simulink model "AMR_main_24a_TesteMobotic"  (R2024a)
settings: Solver=FixedStepAuto  StartTime=0.0  StopTime=inf  FixedStep=1e-3  RelTol=1e-3
model workspace (MAT data in the model file):
  RTK_health_condition = 30
  mdlWSDbList : string (value not decoded)
undefined symbols (not defined in the file or in its folder): Down, Pull
libraries: tramontina_database_nvidialib x11, speedgoatlib_IO60X_IO69X x10, tramontina_database_curtislib x7, tramontina_database_xsenslib x4, tramontina_database_moboticlib x2, speedgoatlib_IO691 x2, canmsglib x1
(part 2 of 2)

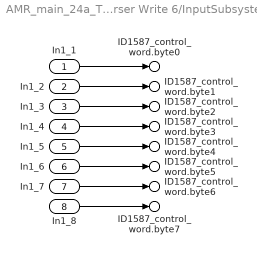
== system AMR_main_24a_TesteMobotic/CAN DB Parser Write 6/InputSubsystem ==
  In1_1 : Inport
  In1_2 : Inport  Port=2
  In1_3 : Inport  Port=3
  In1_4 : Inport  Port=4
  In1_5 : Inport  Port=5
  In1_6 : Inport  Port=6
  In1_7 : Inport  Port=7
  In1_8 : Inport  Port=8
  ID1587_control_word.byte0 : Outport  PortName=OutBus  Element=ID1587_control_word.byte0
  ID1587_control_word.byte1 : Outport  PortName=OutBus  Element=ID1587_control_word.byte1
  ID1587_control_word.byte2 : Outport  PortName=OutBus  Element=ID1587_control_word.byte2
  ID1587_control_word.byte3 : Outport  PortName=OutBus  Element=ID1587_control_word.byte3
  ID1587_control_word.byte4 : Outport  PortName=OutBus  Element=ID1587_control_word.byte4
  ID1587_control_word.byte5 : Outport  PortName=OutBus  Element=ID1587_control_word.byte5
  ID1587_control_word.byte6 : Outport  PortName=OutBus  Element=ID1587_control_word.byte6
  ID1587_control_word.byte7 : Outport  PortName=OutBus  Element=ID1587_control_word.byte7
  wires:
  In1_1/1 -> ID1587_control_word.byte0/1
  In1_2/1 -> ID1587_control_word.byte1/1
  In1_3/1 -> ID1587_control_word.byte2/1
  In1_4/1 -> ID1587_control_word.byte3/1
  In1_5/1 -> ID1587_control_word.byte4/1
  In1_6/1 -> ID1587_control_word.byte5/1
  In1_7/1 -> ID1587_control_word.byte6/1
  In1_8/1 -> ID1587_control_word.byte7/1

== system AMR_main_24a_TesteMobotic/CAN DB Parser Write 6/PackSubsystem ==
  In Bus Element : Inport  PortName=PackIn  Element=ID1587_control_word
  control_word_lib : tramontina_database_moboticlib/CAN pack/control_word  SystemSampleTime=-1  VariantActivationTime=update diagram  AllowFlexibleInterface=on  Latency=0  AutoFrameSizeCalculation=off
  In Bus Element1 : Outport  PortName=PackOut  Element=ID1587_control_word
  wires:
  In Bus Element/1 -> control_word_lib/1
  control_word_lib/1 -> In Bus Element1/1
